simulink model "sm_vehicle_2axle_heave_roll_mu"  (R2025b)
settings: Solver=ode23t  StartTime=0.0  StopTime=14.2  MaxStep=0.2  RelTol=1e-3  AbsTol=1e-3  EnableMultiTasking=on
PostLoadFcn:
  | sm_vehicle_2axle_heave_roll_param
  | sm_vehicle_2axle_heave_roll_scene
  | sm_vehicle_2axle_heave_roll_config_maneuver(bdroot,VehicleData,'plateau');
  | set_param([bdroot '/Vehicle'],'popup_surface_conditions','Checker Right');
StartFcn:
  | tic
StopFcn:
  | Elapsed_Sim_Time = toc;
undefined symbols (not defined in the file): brake_trqTs, Disc, FL, FR, Hydraulic, InitVehicle, Mode, RL, RR, SceneData, valve_maxA, valve_maxO, VehicleData, X, Y, Z
libraries: fl_lib x92, sm_lib x43, nesl_utility x40, sm_vehicle_utilities_lib x21, sdlc_lib x8, SimscapeFluids_lib x8, simulink x2, simulink_extras x1
(part 2 of 5)

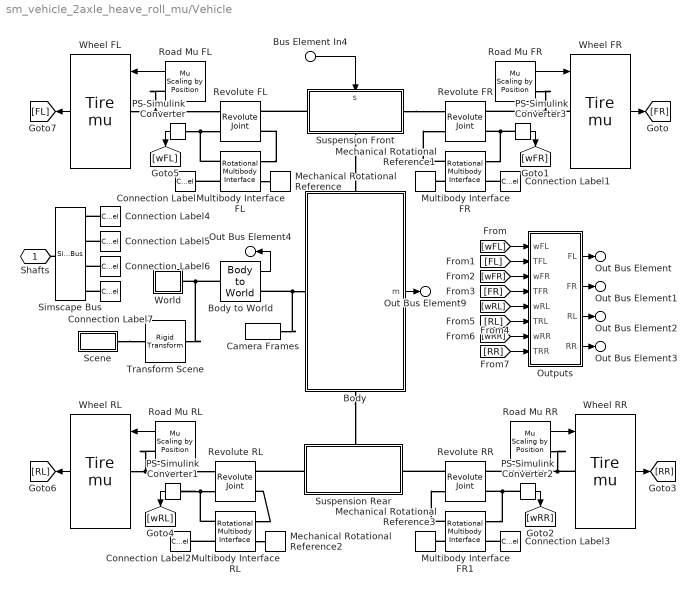
== system sm_vehicle_2axle_heave_roll_mu/Vehicle ==
  Bus Element In4 : Inport  PortName=Drv  Element=sWhl
  Body : Subsystem  mask(Body for 2-Axle Vehicle){xRefToFA=vehdata.Body.FA, xRefToRA=vehdata.Body.RA, xyzRefToCG=vehdata.Body.CG, xyzRefToGeometry=vehdata.Body.Geometry, mBody=vehdata.Body.Mass, JBody=vehdata.Body.Inertias, clrBody=vehdata.Body.Color, opcBody=vehdata.Body.Opacity}
      mask prompts: xRefToFA "Offset Reference to Front Axle (m)"; xRefToRA "Offset Reference to Rear Axle (m)"; xyzRefToCG "Offset Reference to CG [x y z] (m)"; xyzRefToGeometry "Offset Reference to Geometry [x y z] (m)"; mBody "Body Mass (kg)"; JBody "Body Inertia [Ixx Iyy Izz] (kg*m^2)"; clrBody "Body Color [R G B]"; opcBody "Body Opacity (0-1)"
      mask help: Models mass and inertia of rigid vehicle body. Frames for front suspension, rear suspension, center of gravity, and body geometry are all defined relative to the reference frame. Measurements are with respect to the body frame.
      settings: PortSchema="{\"entries\":[{\"content\":{\"sides\":[{\"content\":{\"connectorIds\":[\"LConn1\"]},\"type\":\"ConnectorPlacement.EquallySpacedRectSide\",\"uuid\":\"a6a40084-0b01-416d-a19a-d775fde84bbf\"},{\"content\":{\"connectorIds\":[\"RConn1\"],\"side\":\"RIGHT\"},\"type\":\"ConnectorPlacement.EquallySpacedRectSide\",\"uuid\":\"7b527776-1265-46e3-b587-d37cab880183\"},{\"content\":{\"connectorIds\":[\"Out1\"],\"side\":\"TOP\"},\"type\":\"ConnectorPlacement.EquallySpacedRectSide\",\"uuid\":\"f01e2205-af4e-42ab-b4af-31b005ea0e61\"},{\"content\":{\"connectorIds\":[\"RConn2\"],\"side\":\"BOTTOM\"},\"type\":\"ConnectorPlacement.EquallySpacedRectSide\",\"uuid\":\"682a6e2c-9f3d-4bbb-bb88-e5eb72c2e6bf\"}]},\"type\":\"ConnectorPlacement.EquallySpacedConnector\",\"uuid\":\"a1282978-4c55-459b-9a00-856109b4503f\"}],\"packageUris\":[\"http://schema.mathworks.com/mf0/Connector/R2020b\"],\"version\":\"1.0\"}"
      mask Display: image('sm_vehicle_utilities_body_sedan.png');
  Body to World : sm_vehicle_utilities_lib/Body to World  Init=initveh.Vehicle  SpecifyPosTarget=on
  Camera Frames : sm_vehicle_utilities_lib/Camera Frames  Camera=Camera  popup_dolly_camera=Off
  Connection Label : ConnectionLabel  Label=FL
  Connection Label1 : ConnectionLabel  Label=FR
  Connection Label2 : ConnectionLabel  Label=RL
  Connection Label3 : ConnectionLabel  Label=RR
  Connection Label4 : ConnectionLabel  Label=FL
  Connection Label5 : ConnectionLabel  Label=FR
  Connection Label6 : ConnectionLabel  Label=RL
  Connection Label7 : ConnectionLabel  Label=RR
  Mechanical Rotational Reference{,1..3} (4 alike) : fl_lib/Mechanical/Rotational Elements/Mechanical Rotational Reference
  Multibody Interface FL : fl_lib/Mechanical/Multibody Interfaces/Rotational Multibody Interface
  Multibody Interface FR : fl_lib/Mechanical/Multibody Interfaces/Rotational Multibody Interface
  Multibody Interface FR1 : fl_lib/Mechanical/Multibody Interfaces/Rotational Multibody Interface
  Multibody Interface RL : fl_lib/Mechanical/Multibody Interfaces/Rotational Multibody Interface
  Outputs : Subsystem  mask{whlRadF=vehdata.TireDataF.param.DIMENSION.UNLOADED_RADIUS, whlRadR=vehdata.TireDataR.param.DIMENSION.UNLOADED_RADIUS}
      mask prompts: whlRadF "Wheel Radius Front (m)"; whlRadR "Wheel Radius Rear(m)"
  PS-Simulink Converter{,1..3} (4 alike) : nesl_utility/PS-Simulink Converter  PhysicalDomain=network_engine_domain  SubClassName=ps_output  LeftPortType=input  RightPortType=output  PseudoPeriodic=off  Frequencies=[]  VectorFormat=1-D array  Unit=inherit  AffineConversion=off
  Revolute FL : sm_lib/Joints/Revolute Joint  JointMode=Normal  CompositeWrenchDir=FollowerOnBase  CompositeWrenchFrame=BaseFrame  SenseConstraintForce=off  SenseConstraintTorque=off  SenseTotalForce=off  SenseTotalTorque=off  PositionTargetSpecify=off  PositionTargetPriority=High  PositionTargetValue=0  PositionTargetValueUnits=deg  VelocityTargetSpecify=on  VelocityTargetPriority=High  VelocityTargetValue=initveh.Wheel.wFL  VelocityTargetValueUnits=rad/s  EquilibriumPosition=0  EquilibriumPositionUnits=rad  SpringStiffness=0  SpringStiffnessUnits=N*m/rad  DampingCoefficient=0  DampingCoefficientUnits=N*m/(rad/s)  LowerLimitSpecify=off  LowerLimitBound=-90  LowerLimitBoundUnits=deg  LowerLimitStiffness=1e4  LowerLimitStiffnessUnits=N*m/deg  LowerLimitDamping=10  LowerLimitDampingUnits=N*m/(deg/s)  LowerLimitTransitionRegionWidth=0.1  LowerLimitTransitionRegionWidthUnits=deg  UpperLimitSpecify=off  UpperLimitBound=90  UpperLimitBoundUnits=deg  UpperLimitStiffness=1e4  UpperLimitStiffnessUnits=N*m/deg  UpperLimitDamping=10  UpperLimitDampingUnits=N*m/(deg/s)  UpperLimitTransitionRegionWidth=0.1  UpperLimitTransitionRegionWidthUnits=deg  TorqueActuationMode=InputTorque  MotionActuationMode=ComputedMotion  SensePosition=off  SenseVelocity=on  SenseAcceleration=off  SenseTorqueForce=off  SenseLowerLimitTorqueForce=off  SenseUpperLimitTorqueForce=off
  Revolute FR : sm_lib/Joints/Revolute Joint  JointMode=Normal  CompositeWrenchDir=FollowerOnBase  CompositeWrenchFrame=BaseFrame  SenseConstraintForce=off  SenseConstraintTorque=off  SenseTotalForce=off  SenseTotalTorque=off  PositionTargetSpecify=off  PositionTargetPriority=High  PositionTargetValue=0  PositionTargetValueUnits=deg  VelocityTargetSpecify=on  VelocityTargetPriority=High  VelocityTargetValue=initveh.Wheel.wFR  VelocityTargetValueUnits=rad/s  EquilibriumPosition=0  EquilibriumPositionUnits=rad  SpringStiffness=0  SpringStiffnessUnits=N*m/rad  DampingCoefficient=0  DampingCoefficientUnits=N*m/(rad/s)  LowerLimitSpecify=off  LowerLimitBound=-90  LowerLimitBoundUnits=deg  LowerLimitStiffness=1e4  LowerLimitStiffnessUnits=N*m/deg  LowerLimitDamping=10  LowerLimitDampingUnits=N*m/(deg/s)  LowerLimitTransitionRegionWidth=0.1  LowerLimitTransitionRegionWidthUnits=deg  UpperLimitSpecify=off  UpperLimitBound=90  UpperLimitBoundUnits=deg  UpperLimitStiffness=1e4  UpperLimitStiffnessUnits=N*m/deg  UpperLimitDamping=10  UpperLimitDampingUnits=N*m/(deg/s)  UpperLimitTransitionRegionWidth=0.1  UpperLimitTransitionRegionWidthUnits=deg  TorqueActuationMode=InputTorque  MotionActuationMode=ComputedMotion  SensePosition=off  SenseVelocity=on  SenseAcceleration=off  SenseTorqueForce=off  SenseLowerLimitTorqueForce=off  SenseUpperLimitTorqueForce=off
  Revolute RL : sm_lib/Joints/Revolute Joint  JointMode=Normal  CompositeWrenchDir=FollowerOnBase  CompositeWrenchFrame=BaseFrame  SenseConstraintForce=off  SenseConstraintTorque=off  SenseTotalForce=off  SenseTotalTorque=off  PositionTargetSpecify=off  PositionTargetPriority=High  PositionTargetValue=0  PositionTargetValueUnits=deg  VelocityTargetSpecify=on  VelocityTargetPriority=High  VelocityTargetValue=initveh.Wheel.wRL  VelocityTargetValueUnits=rad/s  EquilibriumPosition=0  EquilibriumPositionUnits=rad  SpringStiffness=0  SpringStiffnessUnits=N*m/rad  DampingCoefficient=0  DampingCoefficientUnits=N*m/(rad/s)  LowerLimitSpecify=off  LowerLimitBound=-90  LowerLimitBoundUnits=deg  LowerLimitStiffness=1e4  LowerLimitStiffnessUnits=N*m/deg  LowerLimitDamping=10  LowerLimitDampingUnits=N*m/(deg/s)  LowerLimitTransitionRegionWidth=0.1  LowerLimitTransitionRegionWidthUnits=deg  UpperLimitSpecify=off  UpperLimitBound=90  UpperLimitBoundUnits=deg  UpperLimitStiffness=1e4  UpperLimitStiffnessUnits=N*m/deg  UpperLimitDamping=10  UpperLimitDampingUnits=N*m/(deg/s)  UpperLimitTransitionRegionWidth=0.1  UpperLimitTransitionRegionWidthUnits=deg  TorqueActuationMode=InputTorque  MotionActuationMode=ComputedMotion  SensePosition=off  SenseVelocity=on  SenseAcceleration=off  SenseTorqueForce=off  SenseLowerLimitTorqueForce=off  SenseUpperLimitTorqueForce=off
  Revolute RR : sm_lib/Joints/Revolute Joint  JointMode=Normal  CompositeWrenchDir=FollowerOnBase  CompositeWrenchFrame=BaseFrame  SenseConstraintForce=off  SenseConstraintTorque=off  SenseTotalForce=off  SenseTotalTorque=off  PositionTargetSpecify=off  PositionTargetPriority=High  PositionTargetValue=0  PositionTargetValueUnits=deg  VelocityTargetSpecify=on  VelocityTargetPriority=High  VelocityTargetValue=initveh.Wheel.wRR  VelocityTargetValueUnits=rad/s  EquilibriumPosition=0  EquilibriumPositionUnits=rad  SpringStiffness=0  SpringStiffnessUnits=N*m/rad  DampingCoefficient=0  DampingCoefficientUnits=N*m/(rad/s)  LowerLimitSpecify=off  LowerLimitBound=-90  LowerLimitBoundUnits=deg  LowerLimitStiffness=1e4  LowerLimitStiffnessUnits=N*m/deg  LowerLimitDamping=10  LowerLimitDampingUnits=N*m/(deg/s)  LowerLimitTransitionRegionWidth=0.1  LowerLimitTransitionRegionWidthUnits=deg  UpperLimitSpecify=off  UpperLimitBound=90  UpperLimitBoundUnits=deg  UpperLimitStiffness=1e4  UpperLimitStiffnessUnits=N*m/deg  UpperLimitDamping=10  UpperLimitDampingUnits=N*m/(deg/s)  UpperLimitTransitionRegionWidth=0.1  UpperLimitTransitionRegionWidthUnits=deg  TorqueActuationMode=InputTorque  MotionActuationMode=ComputedMotion  SensePosition=off  SenseVelocity=on  SenseAcceleration=off  SenseTorqueForce=off  SenseLowerLimitTorqueForce=off  SenseUpperLimitTorqueForce=off
  Road Mu FL : sm_vehicle_utilities_lib/Mu Scaling by Position  mu_out=mu_surface  muP1_in=p1.mu  muP2_in=p2.mu  intvX_P1_start=p1.xstart  intvX_P2_start=p2.xstart  intvX_P1_end=p1.xend  intvX_P2_end=p2.xend  intvY_P1_start=p1.ystart  intvY_P2_start=p2.ystart  intvY_P1_end=p1.yend  intvY_P2_end=p2.yend
  Road Mu FR : sm_vehicle_utilities_lib/Mu Scaling by Position  mu_out=mu_surface  muP1_in=p1.mu  muP2_in=p2.mu  intvX_P1_start=p1.xstart  intvX_P2_start=p2.xstart  intvX_P1_end=p1.xend  intvX_P2_end=p2.xend  intvY_P1_start=p1.ystart  intvY_P2_start=p2.ystart  intvY_P1_end=p1.yend  intvY_P2_end=p2.yend
  Road Mu RL : sm_vehicle_utilities_lib/Mu Scaling by Position  mu_out=mu_surface  muP1_in=p1.mu  muP2_in=p2.mu  intvX_P1_start=p1.xstart  intvX_P2_start=p2.xstart  intvX_P1_end=p1.xend  intvX_P2_end=p2.xend  intvY_P1_start=p1.ystart  intvY_P2_start=p2.ystart  intvY_P1_end=p1.yend  intvY_P2_end=p2.yend
  Road Mu RR : sm_vehicle_utilities_lib/Mu Scaling by Position  mu_out=mu_surface  muP1_in=p1.mu  muP2_in=p2.mu  intvX_P1_start=p1.xstart  intvX_P2_start=p2.xstart  intvX_P1_end=p1.xend  intvX_P2_end=p2.xend  intvY_P1_start=p1.ystart  intvY_P2_start=p2.ystart  intvY_P1_end=p1.yend  intvY_P2_end=p2.yend
  Scene : Subsystem
  Simscape Bus : SimscapeBus  HierarchyStrings=FL;FR;RL;RR
  Suspension Front : Subsystem  mask(Suspension with Heave, Roll, and Ackerman Steering){zHeave=vehdata.SuspF.Heave.Height, kHeave=vehdata.SuspF.Heave.Stiffness, dHeave=vehdata.SuspF.Heave.Damping, xEqHeave=vehdata.SuspF.Heave.EqPos, zRoll=vehdata.SuspF.Roll.Height, kRoll=vehdata.SuspF.Roll.Stiffness, dRoll=vehdata.SuspF.Roll.Damping, aEqRoll=vehdata.SuspF.Roll.EqPos, mUnsprungMass=vehdata.SuspF.UnsprungMass.Mass, JUnsprungMass=vehdata.SuspF.UnsprungMass.Inertia, zUnsprungMass=vehdata.SuspF.UnsprungMass.Height, rUnsprungMass=vehdata.SuspF.UnsprungMass.Radius, lUnsprungMass=vehdata.SuspF.UnsprungMass.Length, zHub=vehdata.SuspF.Hub.Height, yTrack=vehdata.SuspF.Track, wheelbase=sum(abs(vehdata.Body.RA-vehdata.Body.FA)), steerRatio=vehdata.SuspF.SteerRatio}
      mask prompts: zHeave "Height (m)"; kHeave "Stiffness (N/m)"; dHeave "Damping (N/(m/s))"; xEqHeave "Equilibrium Position (m)"; zRoll "Height (m)"; kRoll "Stiffness (N*m/rad)"; dRoll "Damping (N*m/(rad/s)"; aEqRoll "Equilibrium Position (rad)"; mUnsprungMass "Mass (kg)"; JUnsprungMass "Inertia (kg*m^2)"; zUnsprungMass "Height (m)"; rUnsprungMass "Radius (m)"; lUnsprungMass "Length (m)"; zHub "Wheel Center Height (m)"; yTrack "Track Width (m)"; steerRatio "Steering Ratio"
      mask help: Models a suspension with heave and roll degrees of freedom for a single axle, with Ackermann steering. All heights are measured relative to the bottom of the wheels.
      settings: PortSchema="{\"entries\":[{\"content\":{\"sides\":[{\"content\":{\"connectorIds\":[\"LConn1\"]},\"type\":\"ConnectorPlacement.EquallySpacedRectSide\",\"uuid\":\"0af81f34-82de-4f02-a8a7-ec45be82faea\"},{\"content\":{\"connectorIds\":[\"In1\"],\"side\":\"RIGHT\"},\"type\":\"ConnectorPlacement.EquallySpacedRectSide\",\"uuid\":\"9bc48957-2707-4e2f-b988-a5743aaf8f58\"},{\"content\":{\"connectorIds\":[\"LConn2\"],\"side\":\"TOP\"},\"type\":\"ConnectorPlacement.EquallySpacedRectSide\",\"uuid\":\"08055243-2fee-46c8-8a4b-df5231c2978e\"},{\"content\":{\"connectorIds\":[\"RConn1\"],\"side\":\"BOTTOM\"},\"type\":\"ConnectorPlacement.EquallySpacedRectSide\",\"uuid\":\"745b1e5c-9113-4e99-a394-3eadcd3cd6f8\"}]},\"type\":\"ConnectorPlacement.EquallySpacedConnector\",\"uuid\":\"5011d399-f081-425d-a1fb-c00f3859766f\"}],\"packageUris\":[\"http://schema.mathworks.com/mf0/Connector/R2020b\"],\"version\":\"1.0\"}"
      mask DialogControl cont_heave_roll Prompt: Heave, Roll
      mask DialogControl group_heave Prompt: Heave
      mask DialogControl group_roll Prompt: Roll
      mask DialogControl cont_unsprung_mass Prompt: Unsprung Mass
      mask DialogControl cont_wheels_steering Prompt: Wheels, Steering
  Suspension Rear : Subsystem  mask(Suspension with Heave, Roll,){zHeave=vehdata.SuspR.Heave.Height, kHeave=vehdata.SuspR.Heave.Stiffness, dHeave=vehdata.SuspR.Heave.Damping, xEqHeave=vehdata.SuspR.Heave.EqPos, zRoll=vehdata.SuspR.Roll.Height, kRoll=vehdata.SuspR.Roll.Stiffness, dRoll=vehdata.SuspR.Roll.Damping, aEqRoll=vehdata.SuspR.Roll.EqPos, mUnsprungMass=vehdata.SuspR.UnsprungMass.Mass, JUnsprungMass=vehdata.SuspR.UnsprungMass.Inertia, zUnsprungMass=vehdata.SuspR.UnsprungMass.Height, rUnsprungMass=vehdata.SuspR.UnsprungMass.Radius, lUnsprungMass=vehdata.SuspR.UnsprungMass.Length, zHub=vehdata.SuspR.Hub.Height, yTrack=vehdata.SuspR.Track}
      mask prompts: zHeave "Height (m)"; kHeave "Stiffness (N/m)"; dHeave "Damping (N/(m/s))"; xEqHeave "Equilibrium Position (m)"; zRoll "Height (m)"; kRoll "Stiffness (N*m/rad)"; dRoll "Damping (N*m/(rad/s)"; aEqRoll "Equilibrium Position (rad)"; mUnsprungMass "Mass (kg)"; JUnsprungMass "Inertia (kg*m^2)"; zUnsprungMass "Height (m)"; rUnsprungMass "Radius (m)"; lUnsprungMass "Length (m)"; zHub "Wheel Center Height (m)"; yTrack "Track Width (m)"
      mask help: Models a suspension with heave and roll degrees of freedom for a single axle. All heights are measured relative to the bottom of the wheels.
      settings: PortSchema="{\"entries\":[{\"content\":{\"sides\":[{\"content\":{\"connectorIds\":[\"LConn1\"]},\"type\":\"ConnectorPlacement.EquallySpacedRectSide\",\"uuid\":\"0af81f34-82de-4f02-a8a7-ec45be82faea\"},{\"content\":{\"connectorIds\":[],\"side\":\"RIGHT\"},\"type\":\"ConnectorPlacement.EquallySpacedRectSide\",\"uuid\":\"9bc48957-2707-4e2f-b988-a5743aaf8f58\"},{\"content\":{\"connectorIds\":[\"LConn2\"],\"side\":\"TOP\"},\"type\":\"ConnectorPlacement.EquallySpacedRectSide\",\"uuid\":\"08055243-2fee-46c8-8a4b-df5231c2978e\"},{\"content\":{\"connectorIds\":[\"RConn1\"],\"side\":\"BOTTOM\"},\"type\":\"ConnectorPlacement.EquallySpacedRectSide\",\"uuid\":\"3fad50e5-0b96-4492-ad18-fd370deae0ca\"}]},\"type\":\"ConnectorPlacement.EquallySpacedConnector\",\"uuid\":\"5011d399-f081-425d-a1fb-c00f3859766f\"}],\"packageUris\":[\"http://schema.mathworks.com/mf0/Connector/R2020b\"],\"version\":\"1.0\"}"
      mask DialogControl cont_heave_roll Prompt: Heave, Roll
      mask DialogControl group_heave Prompt: Heave
      mask DialogControl group_roll Prompt: Roll
      mask DialogControl cont_unsprung_mass Prompt: Unsprung Mass
      mask DialogControl cont_wheels Prompt: Wheels
  Transform Scene : sm_lib/Frames and Transforms/Rigid Transform  RotationMethod=RotationSequence  FollAlignAxisA=+X  BaseAlignAxisA=+Y  FollAlignAxisB=+Y  BaseAlignAxisB=+Z  RotationStandardAxis=+Y  RotationAngle=0  RotationAngleUnits=deg  RotationArbitraryAxis=[0 0 1]  RotationSequenceAxes=FollowerAxes  RotationSequence=ZYX  RotationSequenceAngles=[SceneData.Reference.yaw SceneData.Reference.pitch SceneData.Reference.roll]  RotationSequenceAnglesUnits=rad  RotationMatrix=[1 0 0; 0 1 0; 0 0 1]  Quaternion=[1 0 0 0]  TranslationMethod=None  TranslationCartesianOffset=[0 0 0]  TranslationCartesianOffsetUnits=m  TranslationStandardAxis=+Z  TranslationStandardOffset=0  TranslationStandardOffsetUnits=m  TranslationROffset=0  TranslationROffsetUnits=m  TranslationThetaOffset=0  TranslationThetaOffsetUnits=deg  TranslationZOffset=0  TranslationZOffsetUnits=m
  Wheel FL : sm_vehicle_utilities_lib/Tire mu  popup_leftright=Left  tire_param=vehdata.TireDataF.param  rim_mass=vehdata.RimF.Mass  rim_inertia=vehdata.RimF.Inertia
  Wheel FR : sm_vehicle_utilities_lib/Tire mu  popup_leftright=Right  tire_param=vehdata.TireDataF.param  rim_mass=vehdata.RimF.Mass  rim_inertia=vehdata.RimF.Inertia
  Wheel RL : sm_vehicle_utilities_lib/Tire mu  popup_leftright=Left  tire_param=vehdata.TireDataR.param  rim_mass=vehdata.RimR.Mass  rim_inertia=vehdata.RimR.Inertia
  Wheel RR : sm_vehicle_utilities_lib/Tire mu  popup_leftright=Right  tire_param=vehdata.TireDataR.param  rim_mass=vehdata.RimR.Mass  rim_inertia=vehdata.RimR.Inertia
  World : Subsystem
  Shafts : PMIOPort  Side=Left
  Out Bus Element9 : Outport  PortName=m  Element=Body
  Out Bus Element : Outport  PortName=m  Element=TireFL
  Out Bus Element1 : Outport  PortName=m  Element=TireFR
  Out Bus Element2 : Outport  PortName=m  Element=TireRL
  Out Bus Element3 : Outport  PortName=m  Element=TireRR
  Out Bus Element4 : Outport  PortName=m  Element=World
  wires:
  Bus Element In4/1 -> Suspension Front/1(s)
  Body/1(m) -> Out Bus Element9/1
  Wheel FL/1 -> [FL]
  Wheel FR/1 -> [FR]
  Wheel RL/1 -> [RL]
  Wheel RR/1 -> [RR]
  Body to World/1 -> Out Bus Element4/1
  Road Mu FL/1 -> Wheel FL/1
  Road Mu FR/1 -> Wheel FR/1
  Road Mu RR/1 -> Wheel RR/1
  Road Mu RL/1 -> Wheel RL/1
  PS-Simulink Converter3/1 -> [wFR]
  PS-Simulink Converter2/1 -> [wRR]
  [wFR] -> Outputs/3(wFR)
  [wRR] -> Outputs/7(wRR)
  [RR] -> Outputs/8(TRR)
  [wRL] -> Outputs/5(wRL)
  [FL] -> Outputs/2(TFL)
  PS-Simulink Converter1/1 -> [wRL]
  [RL] -> Outputs/6(TRL)
  [wFL] -> Outputs/1(wFL)
  [FR] -> Outputs/4(TFR)
  PS-Simulink Converter/1 -> [wFL]
  Outputs/2(FR) -> Out Bus Element1/1
  Outputs/4(RR) -> Out Bus Element3/1
  Outputs/3(RL) -> Out Bus Element2/1
  Outputs/1(FL) -> Out Bus Element/1
  connections:
  Body to World/LConn1 -- Transform Scene/LConn1 -- World/RConn1
  Body/LConn1 -- Suspension Rear/LConn1
  Wheel FR/LConn1 -- Road Mu FR/RConn1 -- Revolute FR/RConn1
  Suspension Front/RConn1 -- Revolute FR/LConn1
  Suspension Front/LConn2 -- Revolute FL/LConn1
  Suspension Rear/LConn2 -- Revolute RL/LConn1
  Revolute RR/LConn1 -- Suspension Rear/RConn1
  Wheel RL/LConn1 -- Revolute RL/RConn1 -- Road Mu RL/RConn1
  Camera Frames/RConn1 -- Body to World/RConn1 -- Body/RConn2
  Wheel FL/LConn1 -- Road Mu FL/RConn1 -- Revolute FL/RConn1
  Wheel RR/LConn1 -- Revolute RR/RConn1 -- Road Mu RR/RConn1
  Suspension Front/LConn1 -- Body/RConn1
  Multibody Interface FR/RConn1 -- PS-Simulink Converter3/LConn1 -- Revolute FR/RConn2
  Multibody Interface FR/LConn1 -- Revolute FR/LConn2
  Multibody Interface FR1/LConn1 -- Revolute RR/LConn2
  Multibody Interface FR1/RConn1 -- Revolute RR/RConn2 -- PS-Simulink Converter2/LConn1
  Multibody Interface RL/LConn1 -- Revolute RL/LConn2
  Multibody Interface RL/RConn1 -- PS-Simulink Converter1/LConn1 -- Revolute RL/RConn2
  Multibody Interface FL/LConn1 -- Revolute FL/LConn2
  Multibody Interface FL/RConn1 -- PS-Simulink Converter/LConn1 -- Revolute FL/RConn2
  Multibody Interface FL/LConn2 -- Mechanical Rotational Reference/LConn1
  Multibody Interface FL/RConn2 -- Connection Label/LConn1
  Multibody Interface FR/LConn2 -- Mechanical Rotational Reference1/LConn1
  Connection Label1/LConn1 -- Multibody Interface FR/RConn2
  Multibody Interface RL/RConn2 -- Connection Label2/LConn1
  Multibody Interface RL/LConn2 -- Mechanical Rotational Reference2/LConn1
  Connection Label3/LConn1 -- Multibody Interface FR1/RConn2
  Multibody Interface FR1/LConn2 -- Mechanical Rotational Reference3/LConn1
  Connection Label4/LConn1 -- Simscape Bus/LConn1
  Connection Label5/LConn1 -- Simscape Bus/LConn2
  Connection Label6/LConn1 -- Simscape Bus/LConn3
  Connection Label7/LConn1 -- Simscape Bus/LConn4
  Simscape Bus/RConn1 -- Shafts/RConn1
  Scene/RConn1 -- Transform Scene/RConn1

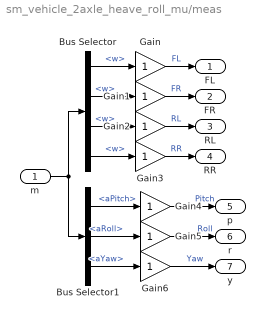
== system sm_vehicle_2axle_heave_roll_mu/meas ==
  m : Inport
  Bus Selector : BusSelector  OutputSignals=TireFL.w,TireFR.w,TireRL.w,TireRR.w
  Bus Selector1 : BusSelector  OutputSignals=Body.aPitch,Body.aRoll,World.aYaw
  Gain{,1..6} (7 alike) : Gain
  FL : Outport
  FR : Outport  Port=2
  RL : Outport  Port=3
  RR : Outport  Port=4
  p : Outport  Port=5
  r : Outport  Port=6
  y : Outport  Port=7
  wires:
  Bus Selector/4 -> Gain3/1  "<w>"
  Bus Selector/2 -> Gain1/1  "<w>"
  Bus Selector/3 -> Gain2/1  "<w>"
  Bus Selector/1 -> Gain/1  "<w>"
  m/1 -> Bus Selector/1, Bus Selector1/1
  Gain3/1 -> RR/1  "RR"
  Gain/1 -> FL/1  "FL"
  Gain1/1 -> FR/1  "FR"
  Gain2/1 -> RL/1  "RL"
  Bus Selector1/1 -> Gain4/1  "<aPitch>"
  Bus Selector1/2 -> Gain5/1  "<aRoll>"
  Bus Selector1/3 -> Gain6/1  "<aYaw>"
  Gain6/1 -> y/1  "Yaw"
  Gain5/1 -> r/1  "Roll"
  Gain4/1 -> p/1  "Pitch"

== system sm_vehicle_2axle_heave_roll_mu/Brakes/Brake Control ==
  Sensor : Inport
  Mode : Subsystem  VariantControl=Mode
  Valve Closed Loop : Subsystem  VariantControl=Valve_Closed_Loop
  Valve Open Loop : Subsystem  VariantControl=Valve_Open_Loop
  " Valves" : Outport  VectorParamsAs1DForOutWhenUnconnected=off

== system sm_vehicle_2axle_heave_roll_mu/Brakes/Brakes ==
  Valve : Inport
  BrkOn : Inport  Port=2
  Damper : Subsystem  VariantControl=Damper  mask(Variable Damper Braking System){max_visc_frict=30*2}
      mask prompts: max_visc_frict "Max Viscous Friction (N/(m/s))"
      mask help: Abstract model of braking system. Brake torque is applied via viscous dampers whose damping coefficient is set by an input signal to mimic varying pressure on the brake pedal. Used to identify amount of torque braking system must provide to slow down the vehicle.
      mask TypeOptions max_visc_frict: Gain FL/Gain | Gain FR/Gain | Gain RL/Gain | Gain RR/Gain
      mask Display: image('sm_vehicle_2axle_brake_damper.png');
  Disc : Subsystem  Tag=PublishSubsystem  VariantControl=Disc  mask(Disc Braking System){actuator_type=Hydraulic, d_caliper_bore_f=0.045, d_caliper_bore_r=0.045}
      mask prompts: actuator_type "Actuator Type"; d_caliper_bore_f "Front Caliper Cylinder Bore (m)"; d_caliper_bore_r "Rear Caliper Cylinder Bore (m)"
      mask help: Disc braking system with configurable actuator. Can configured with ideal force actuators, ideal hydraulic actuators, or valve-driven hydraulic actuators
      mask init:
      | pist_area_pist_f = pi*d_caliper_bore_f^2/4;
      | pist_area_pist_r = pi*d_caliper_bore_r^2/4;
      mask TypeOptions actuator_type: Actuator/actuator_type
      mask Display:
      | act_type = lower(strrep(get_param(gcb,'actuator_type'),' ','_'));
      | 
      | image(['sm_vehicle_2axle_brake_disc_' act_type '.png']);
  " FL" : PMIOPort  Side=Left
  FR : PMIOPort  Port=2  Side=Right
  " RL" : PMIOPort  Port=3  Side=Left
  RR : PMIOPort  Port=4  Side=Right
  " meas" : Outport  VectorParamsAs1DForOutWhenUnconnected=off

== system sm_vehicle_2axle_heave_roll_mu/Brakes/Get Pressure ==
  m : Inport
  Bus Selector2 : BusSelector  OutputSignals=FL.p,FR.p,RL.p,RR.p
  FL : Outport  VectorParamsAs1DForOutWhenUnconnected=off
  FR : Outport  Port=2  VectorParamsAs1DForOutWhenUnconnected=off
  RL : Outport  Port=3  VectorParamsAs1DForOutWhenUnconnected=off
  RR : Outport  Port=4  VectorParamsAs1DForOutWhenUnconnected=off
  wires:
  m/1 -> Bus Selector2/1
  Bus Selector2/4 -> RR/1  "<p>"
  Bus Selector2/1 -> FL/1  "<p>"
  Bus Selector2/2 -> FR/1  "<p>"
  Bus Selector2/3 -> RL/1  "<p>"

== system sm_vehicle_2axle_heave_roll_mu/Brakes/Subsystem ==
  I : Inport
  Bus Creator : BusCreator  Inputs=5
  Bus Creator{1..4} (4 alike) : BusCreator  Inputs=1
  Bus Selector : BusSelector  OutputSignals=Body.vx,TireFL.v,TireFR.v,TireRL.v,TireRR.v
  Gain : Gain
  O : Outport
  wires:
  I/1 -> Bus Selector/1
  Bus Selector/1 -> Gain/1  "<vx>"
  Bus Selector/2 -> Bus Creator1/1  "<v>"
  Bus Selector/3 -> Bus Creator2/1  "<v>"
  Bus Selector/4 -> Bus Creator3/1  "<v>"
  Bus Selector/5 -> Bus Creator4/1  "<v>"
  Bus Creator1/1 -> Bus Creator/2  "FL"
  Bus Creator2/1 -> Bus Creator/3  "FR"
  Bus Creator3/1 -> Bus Creator/4  "RL"
  Bus Creator4/1 -> Bus Creator/5  "RR"
  Gain/1 -> Bus Creator/1  "v"
  Bus Creator/1 -> O/1

== system sm_vehicle_2axle_heave_roll_mu/Driver Input/No Steer ==
  Brake Pedal : Step  Time=0.5  SampleTime=0
  Bus Creator : BusCreator  Inputs=6
  Constant{,1..4} (5 alike) : Constant  Value=0
  Drv : Outport
  wires:
  Constant/1 -> Bus Creator/1  "sWhl"
  Constant3/1 -> Bus Creator/4  "trqRL"
  Constant2/1 -> Bus Creator/3  "trqFR"
  Constant4/1 -> Bus Creator/5  "trqRR"
  Bus Creator/1 -> Drv/1
  Constant1/1 -> Bus Creator/2  "trqFL"
  Brake Pedal/1 -> Bus Creator/6  "BrkPedal"

== system sm_vehicle_2axle_heave_roll_mu/Driver Input/Step Steer ==
  Brake Pedal : Step  Time=0.5  SampleTime=0
  Bus Creator : BusCreator  Inputs=6
  Constant{,1..3} (4 alike) : Constant  Value=0
  Step Steer input : Step  Time=2  After=160*pi/180  SampleTime=0
  Drv : Outport
  wires:
  Step Steer input/1 -> Bus Creator/1  "sWhl"
  Constant2/1 -> Bus Creator/4  "trqRL"
  Constant1/1 -> Bus Creator/3  "trqFR"
  Constant3/1 -> Bus Creator/5  "trqRR"
  Bus Creator/1 -> Drv/1
  Constant/1 -> Bus Creator/2  "trqFL"
  Brake Pedal/1 -> Bus Creator/6  "BrkPedal"

== system sm_vehicle_2axle_heave_roll_mu/Vehicle/Body ==
  Body Inertia : sm_lib/Body Elements/Brick Solid  BrickDimensions=[0.1 0.1 0.1]  BrickDimensionsUnits=m  ExportEntireGeometry=off  InertiaType=Custom  BasedOnType=Density  Density=1000  DensityUnits=kg/(m^3)  Mass=mBody  MassUnits=kg  CenterOfMass=[0 0 0]  CenterOfMassUnits=m  MomentsOfInertia=JBody  MomentsOfInertiaUnits=kg*m^2  ProductsOfInertia=[0 0 0]  ProductsOfInertiaUnits=kg*m^2  GraphicType=FromGeometry  MarkerShape=Sphere  MarkerSize=10  GraphicVisPropType=SimpleVisualProperties  GraphicDiffuseColor=[0.4 0.6 1.0]  GraphicOpacity=1.0  GraphicSpecularColor=[0.5 0.5 0.5 1.0]  GraphicAmbientColor=[0.15 0.15 0.15 1.0]  GraphicEmissiveColor=[0.0 0.0 0.0 1.0]  GraphicShininess=75  DoExposeReferenceFrame=on  SerializedFrames=<Frames/>
  Body Sensor : sm_vehicle_utilities_lib/Body Sensor  offset_body_sensor=[0 0 0]
  Transform CG : sm_lib/Frames and Transforms/Rigid Transform  RotationMethod=None  FollAlignAxisA=+X  BaseAlignAxisA=+Y  FollAlignAxisB=+Y  BaseAlignAxisB=+Z  RotationStandardAxis=+Z  RotationAngle=0  RotationAngleUnits=deg  RotationArbitraryAxis=[0 0 1]  RotationSequenceAxes=FollowerAxes  RotationSequence=XYX  RotationSequenceAngles=[0 0 0]  RotationSequenceAnglesUnits=deg  RotationMatrix=[1 0 0; 0 1 0; 0 0 1]  Quaternion=[1 0 0 0]  TranslationMethod=Cartesian  TranslationCartesianOffset=xyzRefToCG  TranslationCartesianOffsetUnits=m  TranslationStandardAxis=+Z  TranslationStandardOffset=0  TranslationStandardOffsetUnits=m  TranslationROffset=0  TranslationROffsetUnits=m  TranslationThetaOffset=0  TranslationThetaOffsetUnits=deg  TranslationZOffset=0  TranslationZOffsetUnits=m
  Transform Geometry : sm_lib/Frames and Transforms/Rigid Transform  RotationMethod=AlignedAxes  FollAlignAxisA=+Y  BaseAlignAxisA=+Z  FollAlignAxisB=-X  BaseAlignAxisB=+Y  RotationStandardAxis=+Z  RotationAngle=0  RotationAngleUnits=deg  RotationArbitraryAxis=[0 0 1]  RotationSequenceAxes=FollowerAxes  RotationSequence=XYZ  RotationSequenceAngles=[0 0 0]  RotationSequenceAnglesUnits=deg  RotationMatrix=[1 0 0; 0 1 0; 0 0 1]  Quaternion=[1 0 0 0]  TranslationMethod=Cartesian  TranslationCartesianOffset=xyzRefToGeometry  TranslationCartesianOffsetUnits=m  TranslationStandardAxis=+Z  TranslationStandardOffset=0  TranslationStandardOffsetUnits=m  TranslationROffset=0  TranslationROffsetUnits=m  TranslationThetaOffset=0  TranslationThetaOffsetUnits=deg  TranslationZOffset=0  TranslationZOffsetUnits=m
  Transform Suspension Front : sm_lib/Frames and Transforms/Rigid Transform  RotationMethod=None  FollAlignAxisA=+X  BaseAlignAxisA=+Y  FollAlignAxisB=+Y  BaseAlignAxisB=+Z  RotationStandardAxis=+Z  RotationAngle=0  RotationAngleUnits=deg  RotationArbitraryAxis=[0 0 1]  RotationSequenceAxes=FollowerAxes  RotationSequence=XYX  RotationSequenceAngles=[0 0 0]  RotationSequenceAnglesUnits=deg  RotationMatrix=[1 0 0; 0 1 0; 0 0 1]  Quaternion=[1 0 0 0]  TranslationMethod=StandardAxis  TranslationCartesianOffset=[0 0 0]  TranslationCartesianOffsetUnits=m  TranslationStandardAxis=+X  TranslationStandardOffset=xRefToFA  TranslationStandardOffsetUnits=m  TranslationROffset=0  TranslationROffsetUnits=m  TranslationThetaOffset=0  TranslationThetaOffsetUnits=deg  TranslationZOffset=0  TranslationZOffsetUnits=m
  Transform Suspension Rear : sm_lib/Frames and Transforms/Rigid Transform  RotationMethod=None  FollAlignAxisA=+X  BaseAlignAxisA=+Y  FollAlignAxisB=+Y  BaseAlignAxisB=+Z  RotationStandardAxis=+Z  RotationAngle=0  RotationAngleUnits=deg  RotationArbitraryAxis=[0 0 1]  RotationSequenceAxes=FollowerAxes  RotationSequence=XYX  RotationSequenceAngles=[0 0 0]  RotationSequenceAnglesUnits=deg  RotationMatrix=[1 0 0; 0 1 0; 0 0 1]  Quaternion=[1 0 0 0]  TranslationMethod=StandardAxis  TranslationCartesianOffset=[0 0 0]  TranslationCartesianOffsetUnits=m  TranslationStandardAxis=+X  TranslationStandardOffset=xRefToRA  TranslationStandardOffsetUnits=m  TranslationROffset=0  TranslationROffsetUnits=m  TranslationThetaOffset=0  TranslationThetaOffsetUnits=deg  TranslationZOffset=0  TranslationZOffsetUnits=m
  Vehicle Body : sm_lib/Body Elements/File Solid  ExtGeomFileName=sm_vehicle_slalom_vehicle_body.STL  UnitType=Custom  ExtGeomFileUnits=mm  StepReaderType=HEX  ExportConvexHullGeometry=off  InertiaType=Custom  BasedOnType=Density  Density=1000  DensityUnits=kg/m^3  Mass=0.01  MassUnits=kg  CenterOfMass=[0 0 0]  CenterOfMassUnits=m  MomentsOfInertia=[1 1 1]*1e-3  MomentsOfInertiaUnits=kg*m^2  ProductsOfInertia=[0 0 0]  ProductsOfInertiaUnits=kg*m^2  GraphicType=FromGeometry  MarkerShape=Sphere  MarkerSize=10  GraphicVisPropType=SimpleVisualProperties  GraphicDiffuseColor=clrBody  GraphicOpacity=opcBody  GraphicSpecularColor=[0.5 0.5 0.5 1.0]  GraphicAmbientColor=[0.15 0.15 0.15 1.0]  GraphicEmissiveColor=[0.0 0.0 0.0 1.0]  GraphicShininess=75  DoExposeReferenceFrame=on  SerializedFrames=<Frames/>
  RA : PMIOPort  Side=Left
  FA : PMIOPort  Port=2  Side=Right
  Ref : PMIOPort  Port=3  Side=Right
  m : Outport
  wires:
  Body Sensor/1 -> m/1
  connections:
  Transform Suspension Front/RConn1 -- FA/RConn1
  RA/RConn1 -- Transform Suspension Rear/RConn1
  Transform Geometry/RConn1 -- Vehicle Body/RConn1
  Ref/RConn1 -- Transform Suspension Front/LConn1 -- Transform Geometry/LConn1 -- Transform CG/LConn1 -- Transform Suspension Rear/LConn1
  Transform CG/RConn1 -- Body Sensor/LConn1 -- Body Inertia/RConn1

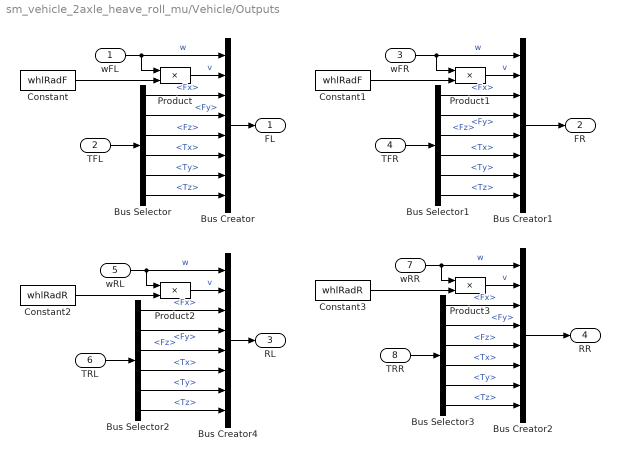
== system sm_vehicle_2axle_heave_roll_mu/Vehicle/Outputs ==
  wFL : Inport
  TFL : Inport  Port=2
  wFR : Inport  Port=3
  TFR : Inport  Port=4
  wRL : Inport  Port=5
  TRL : Inport  Port=6
  wRR : Inport  Port=7
  TRR : Inport  Port=8
  Bus Creator{,1..2,4} (4 alike) : BusCreator  Inputs=8
  Bus Selector{,1..3} (4 alike) : BusSelector  OutputSignals=Fx,Fy,Fz,Tx,Ty,Tz
  Constant : Constant  Value=whlRadF
  Constant1 : Constant  Value=whlRadF
  Constant2 : Constant  Value=whlRadR
  Constant3 : Constant  Value=whlRadR
  Product{,1..3} (4 alike) : Product
  FL : Outport
  FR : Outport  Port=2
  RL : Outport  Port=3
  RR : Outport  Port=4
  wires:
  TFL/1 -> Bus Selector/1
  Bus Selector/1 -> Bus Creator/3  "<Fx>"
  Bus Selector/3 -> Bus Creator/5  "<Fz>"
  Bus Selector/4 -> Bus Creator/6  "<Tx>"
  wFL/1 -> Bus Creator/1, Product/1  "w"
  Bus Selector/2 -> Bus Creator/4  "<Fy>"
  Bus Selector/6 -> Bus Creator/8  "<Tz>"
  Bus Selector/5 -> Bus Creator/7  "<Ty>"
  Bus Creator/1 -> FL/1
  Bus Creator1/1 -> FR/1
  Bus Selector1/5 -> Bus Creator1/7  "<Ty>"
  Bus Selector1/6 -> Bus Creator1/8  "<Tz>"
  Bus Selector1/2 -> Bus Creator1/4  "<Fy>"
  wFR/1 -> Product1/1, Bus Creator1/1  "w"
  Bus Selector1/4 -> Bus Creator1/6  "<Tx>"
  Bus Selector1/3 -> Bus Creator1/5  "<Fz>"
  Bus Selector1/1 -> Bus Creator1/3  "<Fx>"
  TFR/1 -> Bus Selector1/1
  TRR/1 -> Bus Selector3/1
  Bus Selector3/1 -> Bus Creator2/3  "<Fx>"
  Bus Selector3/3 -> Bus Creator2/5  "<Fz>"
  Bus Selector3/4 -> Bus Creator2/6  "<Tx>"
  Bus Selector3/2 -> Bus Creator2/4  "<Fy>"
  Bus Selector3/6 -> Bus Creator2/8  "<Tz>"
  Bus Selector3/5 -> Bus Creator2/7  "<Ty>"
  Bus Creator2/1 -> RR/1
  Bus Creator4/1 -> RL/1
  Bus Selector2/5 -> Bus Creator4/7  "<Ty>"
  Bus Selector2/6 -> Bus Creator4/8  "<Tz>"
  Bus Selector2/2 -> Bus Creator4/4  "<Fy>"
  Bus Selector2/4 -> Bus Creator4/6  "<Tx>"
  Bus Selector2/3 -> Bus Creator4/5  "<Fz>"
  Bus Selector2/1 -> Bus Creator4/3  "<Fx>"
  TRL/1 -> Bus Selector2/1
  Constant/1 -> Product/2
  Product/1 -> Bus Creator/2  "v"
  Product1/1 -> Bus Creator1/2  "v"
  Constant1/1 -> Product1/2
  Product2/1 -> Bus Creator4/2  "v"
  Constant2/1 -> Product2/2
  wRL/1 -> Product2/1, Bus Creator4/1  "w"
  wRR/1 -> Bus Creator2/1, Product3/1  "w"
  Constant3/1 -> Product3/2
  Product3/1 -> Bus Creator2/2  "v"

== system sm_vehicle_2axle_heave_roll_mu/Vehicle/Scene ==
  Grid : Subsystem  VariantControl=Grid  mask{grid_x=SceneData.Grid.length, grid_y=SceneData.Grid.width, grid_z=SceneData.Grid.depth, grid_line_width=SceneData.Grid.linewidth, grid_num_sq_x=SceneData.Grid.numsquaresx, grid_num_sq_y=SceneData.Grid.numsquaresy, grid_clr=SceneData.Grid.linecolor, plane_clr=SceneData.Grid.planecolor, grid_opc=1}
      mask prompts: grid_x "Length (m) (Global x)"; grid_y "Width (m) (Global y)"; grid_z "Depth (m) (Global z)"; grid_line_width "Line width (m)"; grid_num_sq_x "Number of squares in x"; grid_num_sq_y "Number of squares in y"; grid_clr "Line Color [RGB]"; plane_clr "Plane Color [RGB]"; grid_opc "Opacity (0-1)"
      mask init:
      | % Derived parameters - for two perpendicular grids with num_sq-by-1 holes
      | % **Note, not num_sq_x by num_sq_y holes - better render speed with
      | % separate meshes for x and y.
      | 
      | hole_lx = (grid_x-(grid_line_width*(grid_num_sq_x+1)))/grid_num_sq_x;
      | hole_wx = (grid_y-(grid_line_width*(1+1)))/1;
      | 
      | hole_ly = (grid_y-(grid_line_width*(grid_num_sq_y+1)))/grid_num_sq_y;
      | hole_wy = (grid_x-(grid_line_width*(1+1)))/1;
  Patch 1 : sm_lib/Body Elements/Brick Solid  BrickDimensions=p1.dim  BrickDimensionsUnits=m  ExportEntireGeometry=off  InertiaType=CalculateFromGeometry  BasedOnType=Density  Density=1000  DensityUnits=kg/m^3  Mass=1  MassUnits=kg  CenterOfMass=[0 0 0]  CenterOfMassUnits=m  MomentsOfInertia=[1 1 1]  MomentsOfInertiaUnits=kg*m^2  ProductsOfInertia=[0 0 0]  ProductsOfInertiaUnits=kg*m^2  GraphicType=FromGeometry  MarkerShape=Sphere  MarkerSize=10  GraphicVisPropType=SimpleVisualProperties  GraphicDiffuseColor=[0.8 1.0 1.0]  GraphicOpacity=p1.opc  GraphicSpecularColor=[0.5 0.5 0.5 1.0]  GraphicAmbientColor=[0.15 0.15 0.15 1.0]  GraphicEmissiveColor=[0.0 0.0 0.0 1.0]  GraphicShininess=75  DoExposeReferenceFrame=on  SerializedFrames=<Frames/>
  Patch 2 : sm_lib/Body Elements/Brick Solid  BrickDimensions=p2.dim  BrickDimensionsUnits=m  ExportEntireGeometry=off  InertiaType=CalculateFromGeometry  BasedOnType=Density  Density=1000  DensityUnits=kg/m^3  Mass=1  MassUnits=kg  CenterOfMass=[0 0 0]  CenterOfMassUnits=m  MomentsOfInertia=[1 1 1]  MomentsOfInertiaUnits=kg*m^2  ProductsOfInertia=[0 0 0]  ProductsOfInertiaUnits=kg*m^2  GraphicType=FromGeometry  MarkerShape=Sphere  MarkerSize=10  GraphicVisPropType=SimpleVisualProperties  GraphicDiffuseColor=[0.8 1.0 1.0]  GraphicOpacity=p2.opc  GraphicSpecularColor=[0.5 0.5 0.5 1.0]  GraphicAmbientColor=[0.15 0.15 0.15 1.0]  GraphicEmissiveColor=[0.0 0.0 0.0 1.0]  GraphicShininess=75  DoExposeReferenceFrame=on  SerializedFrames=<Frames/>
  Transform Patch 1 : sm_lib/Frames and Transforms/Rigid Transform  RotationMethod=None  FollAlignAxisA=+X  BaseAlignAxisA=+Y  FollAlignAxisB=+Y  BaseAlignAxisB=+Z  RotationStandardAxis=+Z  RotationAngle=0.0  RotationAngleUnits=deg  RotationArbitraryAxis=[0 0 1]  RotationSequenceAxes=FollowerAxes  RotationSequence=XYX  RotationSequenceAngles=[0 0 0]  RotationSequenceAnglesUnits=deg  RotationMatrix=[1 0 0; 0 1 0; 0 0 1]  Quaternion=[1 0 0 0]  TranslationMethod=Cartesian  TranslationCartesianOffset=p1.offset  TranslationCartesianOffsetUnits=m  TranslationStandardAxis=+Z  TranslationStandardOffset=0  TranslationStandardOffsetUnits=m  TranslationROffset=0  TranslationROffsetUnits=m  TranslationThetaOffset=0  TranslationThetaOffsetUnits=deg  TranslationZOffset=0  TranslationZOffsetUnits=m
  Transform Patch 2 : sm_lib/Frames and Transforms/Rigid Transform  RotationMethod=None  FollAlignAxisA=+X  BaseAlignAxisA=+Y  FollAlignAxisB=+Y  BaseAlignAxisB=+Z  RotationStandardAxis=+Z  RotationAngle=0.0  RotationAngleUnits=deg  RotationArbitraryAxis=[0 0 1]  RotationSequenceAxes=FollowerAxes  RotationSequence=XYX  RotationSequenceAngles=[0 0 0]  RotationSequenceAnglesUnits=deg  RotationMatrix=[1 0 0; 0 1 0; 0 0 1]  Quaternion=[1 0 0 0]  TranslationMethod=Cartesian  TranslationCartesianOffset=p2.offset  TranslationCartesianOffsetUnits=m  TranslationStandardAxis=+Z  TranslationStandardOffset=0  TranslationStandardOffsetUnits=m  TranslationROffset=0  TranslationROffsetUnits=m  TranslationThetaOffset=0  TranslationThetaOffsetUnits=deg  TranslationZOffset=0  TranslationZOffsetUnits=m
  B : PMIOPort  Side=Right
  connections:
  Grid/RConn1 -- Transform Patch 1/LConn1 -- Transform Patch 2/LConn1 -- B/RConn1
  Transform Patch 1/RConn1 -- Patch 1/RConn1
  Transform Patch 2/RConn1 -- Patch 2/RConn1
